simulink model "halfcar_tb"  (R2024b)
settings: Solver=VariableStepAuto  StartTime=0.0  StopTime=20  RelTol=1e-3
settings Model: Creator=sebam  LastModifiedBy=sebam

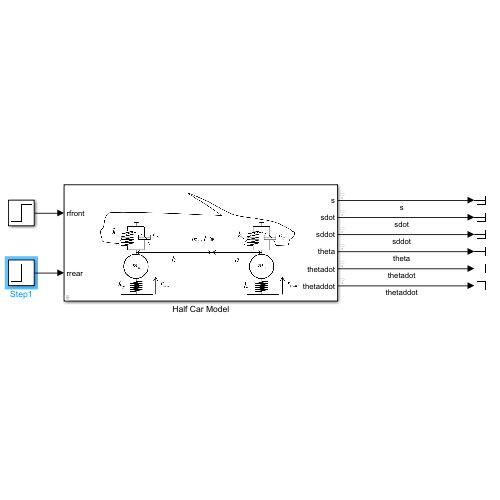
[thumbnail: Simulink's stored preview of the top-level diagram]
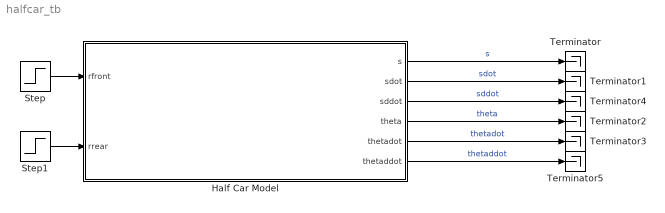
== system halfcar_tb ==
  Half Car Model : Subsystem
      mask Display: image('car.png');
  Step : Step  Time=10  After=0.05  SampleTime=0
  Step1 : Step  Time=15  After=0.05  SampleTime=0
  Terminator{,1..5} (6 alike) : Terminator
  wires:
  Half Car Model/5(thetadot) -> Terminator3/1  "thetadot"
  Half Car Model/4(theta) -> Terminator2/1  "theta"
  Half Car Model/1(s) -> Terminator/1  "s"
  Half Car Model/3(sddot) -> Terminator4/1  "sddot"
  Half Car Model/2(sdot) -> Terminator1/1  "sdot"
  Half Car Model/6(thetaddot) -> Terminator5/1  "thetaddot"
  Step/1 -> Half Car Model/1(rfront)
  Step1/1 -> Half Car Model/2(rrear)

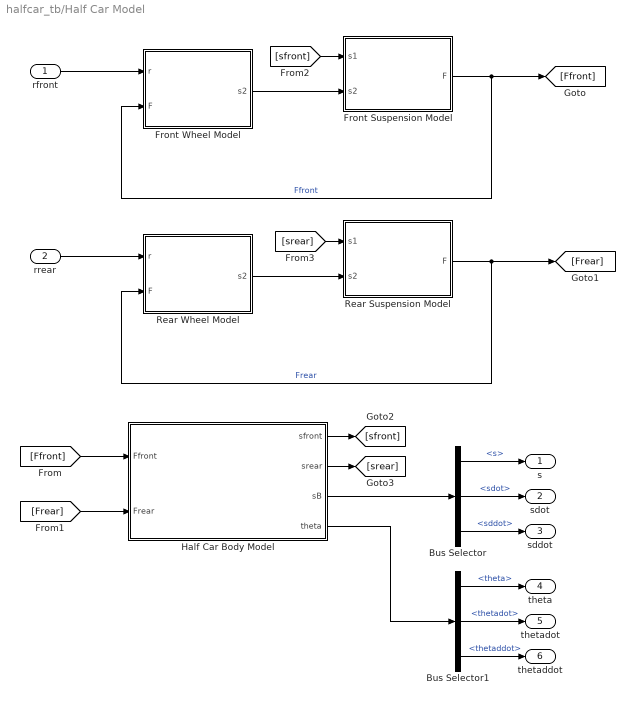
== system halfcar_tb/Half Car Model ==
  rfront : Inport
  rrear : Inport  Port=2
  Bus Selector : BusSelector  OutputSignals=s,sdot,sddot
  Bus Selector1 : BusSelector  OutputSignals=theta,thetadot,thetaddot
  Front Suspension Model : Subsystem  mask{ks=2e4, k2=20*2e4, x0=0.2, ce=1200, cc=600}
      mask prompts: ks "Spring Stiffness (ks)"; k2 "Spring Hardening Stiffness (k2)"; x0 "Spring Hardening Location (x0)"; ce "Damping Rate Extension (cse)"; cc "Damping Rate Compression (csc)"
      settings: AttributesFormatString=|
      | ks = %<ks>
      | k2 = %<k2>
      | x0 = %<x0>
      | ce = %<ce>
      | cc = %<cc>
      mask Display: fprintf("Suspension\nModel")
  Front Wheel Model : Subsystem  mask{m2=20, g=9.81, kT=14e4}
      mask prompts: m2 "Mass (m2)"; g "Gravity (g)"; kT "Wheel Stiffness (kT)"
      settings: AttributesFormatString=|
      | g = %<g>
      | kT = %<kT>
      | m2 = %<m2>
      mask Display: fprintf("Wheel\nModel")
  Half Car Body Model : Subsystem  mask{mB=700, IB=650, g=9.81, a=1.35, b=1.5}
      mask prompts: mB "Mass (mB)"; IB "Moment of Inertia (IB)"; g "Gravity (g)"; a "Length A (a)"; b "Length B (b)"
      settings: AttributesFormatString=|
      | mB = %<mB>
      | IB = %<IB>
      | g = %<g>
      | a = %<a>
      | b = %<b>
      mask Display: fprintf("Half Car\nBody Model")
  Rear Suspension Model : Subsystem  mask{ks=2e4, k2=20*2e4, x0=0.2, ce=1200, cc=600}
      mask prompts: ks "Spring Stiffness (ks)"; k2 "Spring Hardening Stiffness (k2)"; x0 "Spring Hardening Location (x0)"; ce "Damping Rate Extension (cse)"; cc "Damping Rate Compression (csc)"
      settings: AttributesFormatString=|
      | ks = %<ks>
      | k2 = %<k2>
      | x0 = %<x0>
      | ce = %<ce>
      | cc = %<cc>
      mask Display: fprintf("Suspension\nModel")
  Rear Wheel Model : Subsystem  mask{m2=20, g=9.81, kT=14e4}
      mask prompts: m2 "Mass (m2)"; g "Gravity (g)"; kT "Wheel Stiffness (kT)"
      settings: AttributesFormatString=|
      | g = %<g>
      | kT = %<kT>
      | m2 = %<m2>
      mask Display: fprintf("Wheel\nModel")
  s : Outport
  sdot : Outport  Port=2
  sddot : Outport  Port=3
  theta : Outport  Port=4
  thetadot : Outport  Port=5
  thetaddot : Outport  Port=6
  wires:
  Front Wheel Model/1(s2) -> Front Suspension Model/2(s2)
  Half Car Body Model/3(sB) -> Bus Selector/1
  Front Suspension Model/1(F) -> [Ffront], Front Wheel Model/2(F)  "Ffront"
  Bus Selector/2 -> sdot/1  "<sdot>"
  Half Car Body Model/4(theta) -> Bus Selector1/1
  Bus Selector1/1 -> theta/1  "<theta>"
  rfront/1 -> Front Wheel Model/1(r)
  Bus Selector1/2 -> thetadot/1  "<thetadot>"
  rrear/1 -> Rear Wheel Model/1(r)
  Bus Selector/1 -> s/1  "<s>"
  Rear Suspension Model/1(F) -> [Frear], Rear Wheel Model/2(F)  "Frear"
  Rear Wheel Model/1(s2) -> Rear Suspension Model/2(s2)
  [Ffront] -> Half Car Body Model/1(Ffront)
  [Frear] -> Half Car Body Model/2(Frear)
  Half Car Body Model/1(sfront) -> [sfront]
  Half Car Body Model/2(srear) -> [srear]
  [sfront] -> Front Suspension Model/1(s1)
  [srear] -> Rear Suspension Model/1(s1)
  Bus Selector/3 -> sddot/1  "<sddot>"
  Bus Selector1/3 -> thetaddot/1  "<thetaddot>"

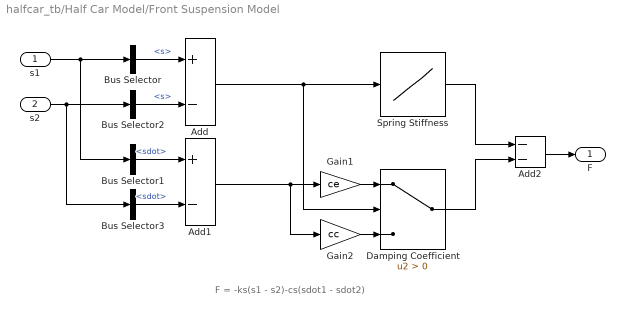
== system halfcar_tb/Half Car Model/Front Suspension Model ==
  note: F = -ks(s1 - s2)-cs(sdot1 - sdot2)
  s1 : Inport
  s2 : Inport  Port=2
  Add : Sum  Inputs=+-
  Add1 : Sum  Inputs=+-
  Add2 : Sum  Inputs=--
  Bus Selector : BusSelector  OutputSignals=s
  Bus Selector1 : BusSelector  OutputSignals=sdot
  Bus Selector2 : BusSelector  OutputSignals=s
  Bus Selector3 : BusSelector  OutputSignals=sdot
  Damping Coefficient : Switch  Criteria=u2 > Threshold  SaturateOnIntegerOverflow=off  InputSameDT=off
  Gain1 : Gain  Gain=ce
  Gain2 : Gain  Gain=cc
  Spring Stiffness : Lookup_n-D  NumberOfTableDimensions=1  BreakpointsForDimension1=[-2*x0, -x0, x0, 2*x0]  Table=[-(ks+k2)*x0, -ks*x0, ks*x0, (ks+k2)*x0]  InternalRulePriority=Speed  RndMeth=Simplest
  F : Outport
  wires:
  s1/1 -> Bus Selector1/1, Bus Selector/1
  s2/1 -> Bus Selector2/1, Bus Selector3/1
  Add/1 -> Spring Stiffness/1, Damping Coefficient/2
  Bus Selector/1 -> Add/1  "<s>"
  Bus Selector1/1 -> Add1/1  "<sdot>"
  Add1/1 -> Gain2/1, Gain1/1
  Spring Stiffness/1 -> Add2/1
  Damping Coefficient/1 -> Add2/2
  Add2/1 -> F/1
  Bus Selector2/1 -> Add/2  "<s>"
  Bus Selector3/1 -> Add1/2  "<sdot>"
  Gain1/1 -> Damping Coefficient/1
  Gain2/1 -> Damping Coefficient/3

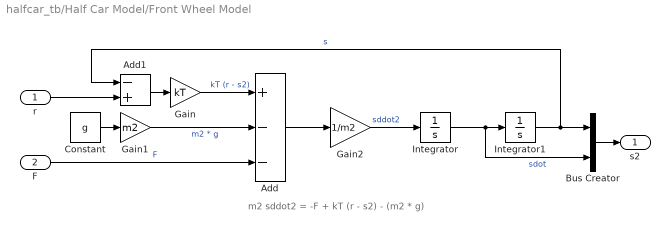
== system halfcar_tb/Half Car Model/Front Wheel Model ==
  note: m2 sddot2 = -F + kT (r - s2) - (m2 * g)
  r : Inport
  F : Inport  Port=2
  Add : Sum  Inputs=+--
  Add1 : Sum  Inputs=-+
  Bus Creator : BusCreator  Inputs=2
  Constant : Constant  Value=g
  Gain : Gain  Gain=kT
  Gain1 : Gain  Gain=m2
  Gain2 : Gain  Gain=1/m2
  Integrator : Integrator
  Integrator1 : Integrator
  s2 : Outport
  wires:
  r/1 -> Add1/2
  Bus Creator/1 -> s2/1
  Gain2/1 -> Integrator/1  "sddot2"
  Constant/1 -> Gain1/1
  Integrator/1 -> Bus Creator/2, Integrator1/1  "sdot"
  Add/1 -> Gain2/1
  Integrator1/1 -> Add1/1, Bus Creator/1  "s"
  Gain1/1 -> Add/2  "m2 * g"
  F/1 -> Add/3  "F"
  Gain/1 -> Add/1  "kT (r - s2)"
  Add1/1 -> Gain/1

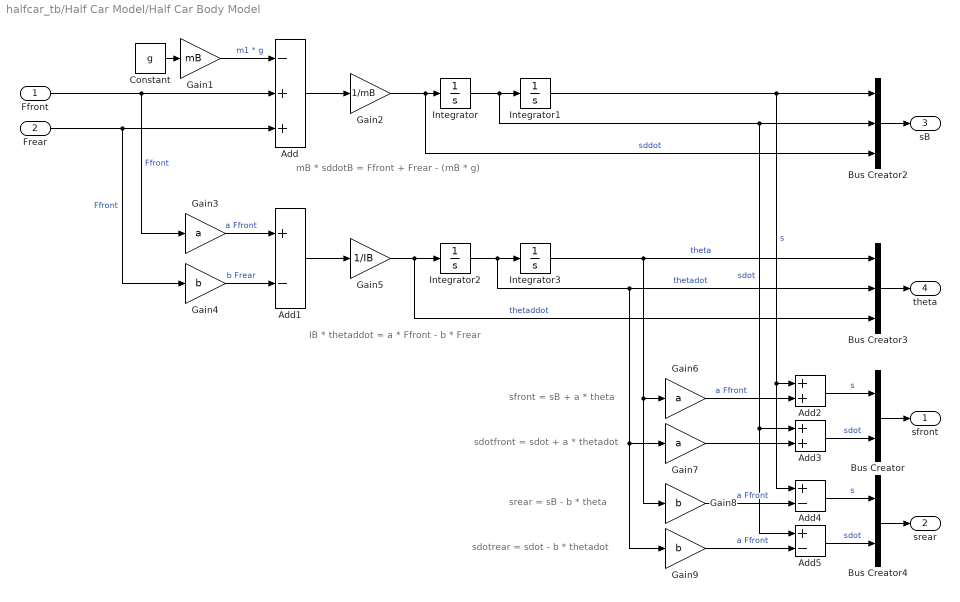
== system halfcar_tb/Half Car Model/Half Car Body Model ==
  note: sfront = sB + a * theta
  note: IB * thetaddot = a * Ffront - b * Frear
  note: mB * sddotB = Ffront + Frear - (mB * g)
  note: sdotfront = sdot + a * thetadot
  note: srear = sB - b * theta
  note: sdotrear = sdot - b * thetadot
  Ffront : Inport
  Frear : Inport  Port=2
  Add : Sum  Inputs=-++
  Add1 : Sum  Inputs=+-
  Add2 : Sum
  Add3 : Sum
  Add4 : Sum  Inputs=+-
  Add5 : Sum  Inputs=+-
  Bus Creator : BusCreator  Inputs=2
  Bus Creator2 : BusCreator  Inputs=3
  Bus Creator3 : BusCreator  Inputs=3
  Bus Creator4 : BusCreator  Inputs=2
  Constant : Constant  Value=g
  Gain1 : Gain  Gain=mB
  Gain2 : Gain  Gain=1/mB
  Gain3 : Gain  Gain=a
  Gain4 : Gain  Gain=b
  Gain5 : Gain  Gain=1/IB
  Gain6 : Gain  Gain=a
  Gain7 : Gain  Gain=a
  Gain8 : Gain  Gain=b
  Gain9 : Gain  Gain=b
  Integrator{,1..3} (4 alike) : Integrator
  sfront : Outport
  srear : Outport  Port=2
  sB : Outport  Port=3
  theta : Outport  Port=4
  wires:
  Integrator1/1 -> Add4/1, Add2/1, Bus Creator2/1  "s"
  Add/1 -> Gain2/1
  Constant/1 -> Gain1/1
  Gain1/1 -> Add/1  "m1 * g"
  Gain2/1 -> Bus Creator2/3, Integrator/1  "sddot"
  Bus Creator/1 -> sfront/1
  Bus Creator4/1 -> srear/1
  Bus Creator2/1 -> sB/1
  Integrator/1 -> Integrator1/1, Add5/1, Add3/1, Bus Creator2/2  "sdot"
  Add3/1 -> Bus Creator/2  "sdot"
  Gain3/1 -> Add1/1  "a Ffront"
  Gain4/1 -> Add1/2  "b Frear"
  Add1/1 -> Gain5/1
  Gain5/1 -> Bus Creator3/3, Integrator2/1  "thetaddot"
  Integrator2/1 -> Gain9/1, Gain7/1, Bus Creator3/2, Integrator3/1  "thetadot"
  Integrator3/1 -> Gain8/1, Gain6/1, Bus Creator3/1  "theta"
  Bus Creator3/1 -> theta/1
  Add2/1 -> Bus Creator/1  "s"
  Gain6/1 -> Add2/2  "a Ffront"
  Gain7/1 -> Add3/2
  Add4/1 -> Bus Creator4/1  "s"
  Add5/1 -> Bus Creator4/2  "sdot"
  Gain8/1 -> Add4/2  "a Ffront"
  Gain9/1 -> Add5/2  "a Ffront"
  Ffront/1 -> Gain3/1, Add/2  "Ffront"
  Frear/1 -> Gain4/1, Add/3  "Ffront"

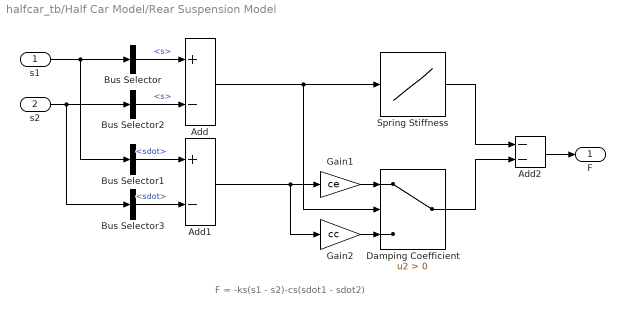
== system halfcar_tb/Half Car Model/Rear Suspension Model ==
  note: F = -ks(s1 - s2)-cs(sdot1 - sdot2)
  s1 : Inport
  s2 : Inport  Port=2
  Add : Sum  Inputs=+-
  Add1 : Sum  Inputs=+-
  Add2 : Sum  Inputs=--
  Bus Selector : BusSelector  OutputSignals=s
  Bus Selector1 : BusSelector  OutputSignals=sdot
  Bus Selector2 : BusSelector  OutputSignals=s
  Bus Selector3 : BusSelector  OutputSignals=sdot
  Damping Coefficient : Switch  Criteria=u2 > Threshold  SaturateOnIntegerOverflow=off  InputSameDT=off
  Gain1 : Gain  Gain=ce
  Gain2 : Gain  Gain=cc
  Spring Stiffness : Lookup_n-D  NumberOfTableDimensions=1  BreakpointsForDimension1=[-2*x0, -x0, x0, 2*x0]  Table=[-(ks+k2)*x0, -ks*x0, ks*x0, (ks+k2)*x0]  InternalRulePriority=Speed  RndMeth=Simplest
  F : Outport
  wires:
  Damping Coefficient/1 -> Add2/2
  Add1/1 -> Gain2/1, Gain1/1
  Add2/1 -> F/1
  Bus Selector/1 -> Add/1  "<s>"
  Bus Selector2/1 -> Add/2  "<s>"
  Bus Selector1/1 -> Add1/1  "<sdot>"
  Bus Selector3/1 -> Add1/2  "<sdot>"
  s2/1 -> Bus Selector2/1, Bus Selector3/1
  Gain2/1 -> Damping Coefficient/3
  s1/1 -> Bus Selector1/1, Bus Selector/1
  Gain1/1 -> Damping Coefficient/1
  Add/1 -> Spring Stiffness/1, Damping Coefficient/2
  Spring Stiffness/1 -> Add2/1

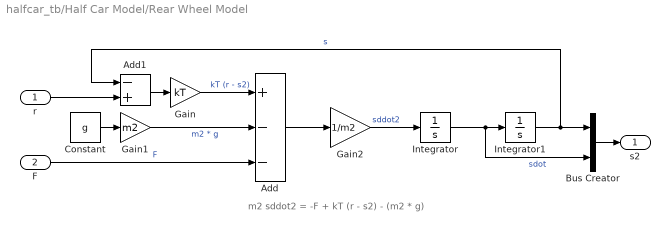
== system halfcar_tb/Half Car Model/Rear Wheel Model ==
  note: m2 sddot2 = -F + kT (r - s2) - (m2 * g)
  r : Inport
  F : Inport  Port=2
  Add : Sum  Inputs=+--
  Add1 : Sum  Inputs=-+
  Bus Creator : BusCreator  Inputs=2
  Constant : Constant  Value=g
  Gain : Gain  Gain=kT
  Gain1 : Gain  Gain=m2
  Gain2 : Gain  Gain=1/m2
  Integrator : Integrator
  Integrator1 : Integrator
  s2 : Outport
  wires:
  Add1/1 -> Gain/1
  Gain/1 -> Add/1  "kT (r - s2)"
  F/1 -> Add/3  "F"
  Gain1/1 -> Add/2  "m2 * g"
  Integrator1/1 -> Bus Creator/1, Add1/1  "s"
  Add/1 -> Gain2/1
  Integrator/1 -> Integrator1/1, Bus Creator/2  "sdot"
  Constant/1 -> Gain1/1
  Gain2/1 -> Integrator/1  "sddot2"
  Bus Creator/1 -> s2/1
  r/1 -> Add1/2
